simulink model "SMCextended"  (R2020b)
settings: Solver=VariableStepAuto  StartTime=0.0  StopTime=10.0  RelTol=1e-3
undefined symbols (not defined in the file): b, delta, g, Kc, l, m
settings Model: Creator=andre  LastModifiedBy=andre

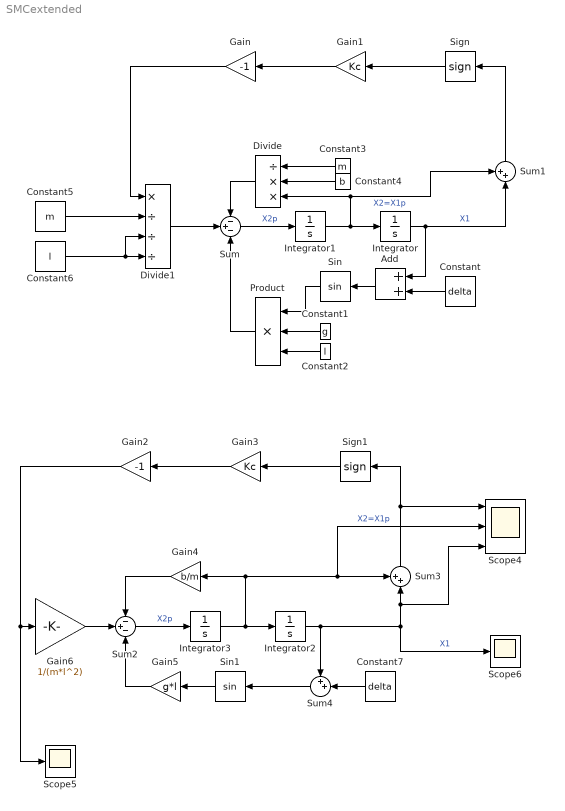
== system SMCextended ==
  Add : Sum
  Constant : Constant  Value=delta
  Constant1 : Constant  Value=g
  Constant2 : Constant  Value=l
  Constant3 : Constant  Value=m
  Constant4 : Constant  Value=b
  Constant5 : Constant  Value=m
  Constant6 : Constant  Value=l
  Constant7 : Constant  Value=delta
  Divide : Product  Inputs=/**
  Divide1 : Product  Inputs=*///
  Gain : Gain  Gain=-1
  Gain1 : Gain  Gain=Kc
  Gain2 : Gain  Gain=-1
  Gain3 : Gain  Gain=Kc
  Gain4 : Gain  Gain=b/m
  Gain5 : Gain  Gain=g*l
  Gain6 : Gain  Gain=1/(m*l^2)
  Integrator{,1..3} (4 alike) : Integrator
  Product : Product  Inputs=3
  Scope4 : Scope  NumInputPorts=3
  Scope5 : Scope
  Scope6 : Scope
  Sign : Signum  ZeroCross=off
  Sign1 : Signum  ZeroCross=off
  Sin : Trigonometry
  Sin1 : Trigonometry
  Sum : Sum  Inputs=-+-
  Sum1 : Sum  Inputs=++|
  Sum2 : Sum  Inputs=-+-
  Sum3 : Sum  Inputs=++|
  Sum4 : Sum  Inputs=++|
  wires:
  Integrator1/1 -> Sum1/1, Divide/3, Integrator/1  "X2=X1p"
  Integrator/1 -> Sum1/2, Add/1  "X1"
  Sum/1 -> Integrator1/1  "X2p"
  Add/1 -> Sin/1
  Constant/1 -> Add/2
  Sin/1 -> Product/1
  Constant1/1 -> Product/2
  Constant2/1 -> Product/3
  Product/1 -> Sum/3
  Constant3/1 -> Divide/1
  Constant4/1 -> Divide/2
  Divide/1 -> Sum/1
  Divide1/1 -> Sum/2
  Constant5/1 -> Divide1/2
  Constant6/1 -> Divide1/4, Divide1/3
  Sum1/1 -> Sign/1
  Sign/1 -> Gain1/1
  Gain1/1 -> Gain/1
  Gain/1 -> Divide1/1
  Gain2/1 -> Scope5/1, Gain6/1
  Sum2/1 -> Integrator3/1  "X2p"
  Sum3/1 -> Sign1/1, Scope4/1
  Gain4/1 -> Sum2/1
  Sin1/1 -> Gain5/1
  Integrator2/1 -> Scope4/3, Sum3/2, Scope6/1, Sum4/1  "X1"
  Gain5/1 -> Sum2/3
  Integrator3/1 -> Gain4/1, Scope4/2, Sum3/1, Integrator2/1  "X2=X1p"
  Constant7/1 -> Sum4/2
  Gain6/1 -> Sum2/2
  Sum4/1 -> Sin1/1
  Gain3/1 -> Gain2/1
  Sign1/1 -> Gain3/1
